simulink library "ScopeHandler"  (R2016b)
settings: Solver=VariableStepAuto  StartTime=0.0  StopTime=10.0  RelTol=1e-3
libraries: ConversionsLibrary x16, slrtlib x9, VariousLibrary x6
settings Model: Creator=Nathan  LastModifiedBy=march

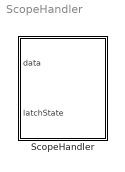
== system ScopeHandler ==
  ScopeHandler : Subsystem

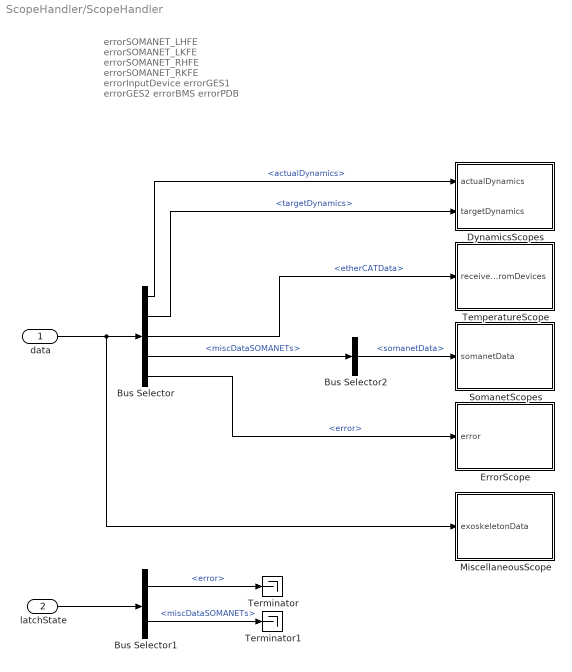
== system ScopeHandler/ScopeHandler ==
  note: errorSOMANET_LHFE
      | errorSOMANET_LKFE
      | errorSOMANET_RHFE
      | errorSOMANET_RKFE
      | errorInputDevice
      | errorGES1
      | errorGES2
      | errorBMS
      | errorPDB
  data : Inport  OutDataTypeStr=Bus: ExoskeletonData  BusOutputAsStruct=on
  latchState : Inport  Port=2  OutDataTypeStr=Bus: ExoskeletonData  BusOutputAsStruct=on
  Bus Selector : BusSelector  OutputSignals=actualDynamics,targetDynamics,etherCATData,miscDataSOMANETs,error
  Bus Selector1 : BusSelector  OutputSignals=error,miscDataSOMANETs
  Bus Selector2 : BusSelector  OutputSignals=somanetData
  DynamicsScopes : Subsystem
  ErrorScope : Subsystem
  MiscellaneousScope : Subsystem
  SomanetScopes : Subsystem
  TemperatureScope : Subsystem
  Terminator : Terminator
  Terminator1 : Terminator
  wires:
  Bus Selector2/1 -> SomanetScopes/1(somanetData)  "<somanetData>"
  Bus Selector/3 -> TemperatureScope/1(receivedFromDevices)  "<etherCATData>"
  Bus Selector/2 -> DynamicsScopes/2(targetDynamics)  "<targetDynamics>"
  Bus Selector/1 -> DynamicsScopes/1(actualDynamics)  "<actualDynamics>"
  Bus Selector/4 -> Bus Selector2/1  "<miscDataSOMANETs>"
  Bus Selector1/2 -> Terminator1/1  "<miscDataSOMANETs>"
  Bus Selector1/1 -> Terminator/1  "<error>"
  Bus Selector/5 -> ErrorScope/1(error)  "<error>"
  data/1 -> Bus Selector/1, MiscellaneousScope/1(exoskeletonData)
  latchState/1 -> Bus Selector1/1

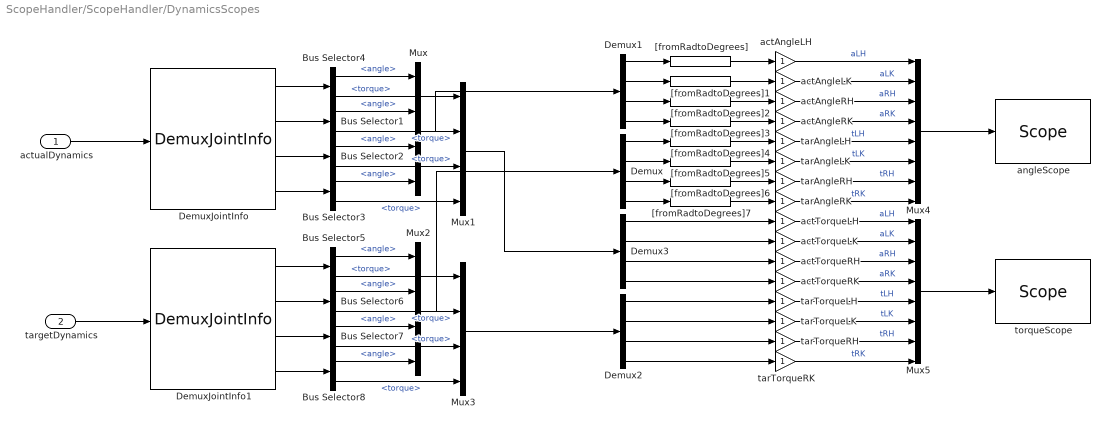
== system ScopeHandler/ScopeHandler/DynamicsScopes ==
  actualDynamics : Inport
  targetDynamics : Inport  Port=2
  Bus Selector{1..8} (8 alike) : BusSelector  OutputSignals=angle,torque
  Demux{,1..3} (4 alike) : Demux
  DemuxJointInfo : VariousLibrary/DemuxJointInfo
  DemuxJointInfo1 : VariousLibrary/DemuxJointInfo
  Mux{,1..3} (4 alike) : Mux
  Mux4 : Mux  Inputs=8
  Mux5 : Mux  Inputs=8
  [fromRadtoDegrees]{,1..7} (8 alike) : ConversionsLibrary/[fromRadtoDegrees]
  actAngleLH : Gain
  actAngleLK : Gain
  actAngleRH : Gain
  actAngleRK : Gain
  actTorqueLH : Gain
  actTorqueLK : Gain
  actTorqueRH : Gain
  actTorqueRK : Gain
  angleScope : slrtlib/Displays and Logging/Scope   scopeno=1  scopetype=Target  autostart=on  viewmode=Graphical rolling  formatstr='%15.6f'  grid=on  ylimits=[-180,180]  nosamples=2000  noprepostsamples=0  interleave=1  triggermode=FreeRun  triggersignal=1  trigsignalfromport=off  triggerlevel=0.0  triggerslope=Either  triggerscope=1  triggersample=0  filename=data.dat  mode=Lazy  writesize=512  autorestart=off  dynamicfilemode=off  maxwritefilesize=512*1024^2
  tarAngleLH : Gain
  tarAngleLK : Gain
  tarAngleRH : Gain
  tarAngleRK : Gain
  tarTorqueLH : Gain
  tarTorqueLK : Gain
  tarTorqueRH : Gain
  tarTorqueRK : Gain
  "torqueScope " : slrtlib/Displays and Logging/Scope   scopeno=2  scopetype=Target  autostart=on  viewmode=Graphical rolling  formatstr='%15.6f'  grid=on  ylimits=[-2.4,2.4]  nosamples=250  noprepostsamples=0  interleave=1  triggermode=FreeRun  triggersignal=1  trigsignalfromport=off  triggerlevel=0.0  triggerslope=Either  triggerscope=1  triggersample=0  filename=data.dat  mode=Lazy  writesize=512  autorestart=off  dynamicfilemode=off  maxwritefilesize=512*1024^2
  wires:
  Mux5/1 -> "torqueScope "/1
  Mux4/1 -> angleScope/1
  "[fromRadtoDegrees]7"/1 -> tarAngleRK/1
  "[fromRadtoDegrees]6"/1 -> tarAngleRH/1
  "[fromRadtoDegrees]5"/1 -> tarAngleLK/1
  "[fromRadtoDegrees]4"/1 -> tarAngleLH/1
  "[fromRadtoDegrees]3"/1 -> actAngleRK/1
  "[fromRadtoDegrees]2"/1 -> actAngleRH/1
  "[fromRadtoDegrees]1"/1 -> actAngleLK/1
  "[fromRadtoDegrees]"/1 -> actAngleLH/1
  tarTorqueRH/1 -> Mux5/7  "tRH"
  tarTorqueLK/1 -> Mux5/6  "tLK"
  tarTorqueLH/1 -> Mux5/5  "tLH"
  tarTorqueRK/1 -> Mux5/8  "tRK"
  Demux2/2 -> tarTorqueLK/1
  Demux2/1 -> tarTorqueLH/1
  Demux2/4 -> tarTorqueRK/1
  Demux2/3 -> tarTorqueRH/1
  actTorqueRK/1 -> Mux5/4  "aRK"
  actTorqueRH/1 -> Mux5/3  "aRH"
  actTorqueLK/1 -> Mux5/2  "aLK"
  actTorqueLH/1 -> Mux5/1  "aLH"
  Demux3/4 -> actTorqueRK/1
  Demux3/2 -> actTorqueLK/1
  Demux3/3 -> actTorqueRH/1
  Demux3/1 -> actTorqueLH/1
  tarAngleRK/1 -> Mux4/8  "tRK"
  tarAngleLH/1 -> Mux4/5  "tLH"
  tarAngleLK/1 -> Mux4/6  "tLK"
  tarAngleRH/1 -> Mux4/7  "tRH"
  Demux/2 -> "[fromRadtoDegrees]5"/1
  Demux/1 -> "[fromRadtoDegrees]4"/1
  Demux/3 -> "[fromRadtoDegrees]6"/1
  Demux/4 -> "[fromRadtoDegrees]7"/1
  actAngleRH/1 -> Mux4/3  "aRH"
  actAngleLH/1 -> Mux4/1  "aLH"
  actAngleLK/1 -> Mux4/2  "aLK"
  actAngleRK/1 -> Mux4/4  "aRK"
  Demux1/4 -> "[fromRadtoDegrees]3"/1
  Demux1/3 -> "[fromRadtoDegrees]2"/1
  Demux1/1 -> "[fromRadtoDegrees]"/1
  Demux1/2 -> "[fromRadtoDegrees]1"/1
  Mux3/1 -> Demux2/1
  Mux1/1 -> Demux3/1
  Mux2/1 -> Demux/1
  Mux/1 -> Demux1/1
  Bus Selector8/2 -> Mux3/4  "<torque>"
  Bus Selector8/1 -> Mux2/4  "<angle>"
  Bus Selector7/2 -> Mux3/3  "<torque>"
  Bus Selector7/1 -> Mux2/3  "<angle>"
  Bus Selector6/2 -> Mux3/2  "<torque>"
  Bus Selector6/1 -> Mux2/2  "<angle>"
  Bus Selector5/2 -> Mux3/1  "<torque>"
  Bus Selector5/1 -> Mux2/1  "<angle>"
  Bus Selector3/2 -> Mux1/4  "<torque>"
  Bus Selector3/1 -> Mux/4  "<angle>"
  Bus Selector2/2 -> Mux1/3  "<torque>"
  Bus Selector2/1 -> Mux/3  "<angle>"
  Bus Selector1/2 -> Mux1/2  "<torque>"
  Bus Selector1/1 -> Mux/2  "<angle>"
  Bus Selector4/2 -> Mux1/1  "<torque>"
  Bus Selector4/1 -> Mux/1  "<angle>"
  DemuxJointInfo1/3 -> Bus Selector7/1
  DemuxJointInfo1/4 -> Bus Selector8/1
  DemuxJointInfo1/1 -> Bus Selector5/1
  DemuxJointInfo1/2 -> Bus Selector6/1
  DemuxJointInfo/3 -> Bus Selector2/1
  DemuxJointInfo/1 -> Bus Selector4/1
  DemuxJointInfo/4 -> Bus Selector3/1
  DemuxJointInfo/2 -> Bus Selector1/1
  targetDynamics/1 -> DemuxJointInfo1/1
  actualDynamics/1 -> DemuxJointInfo/1

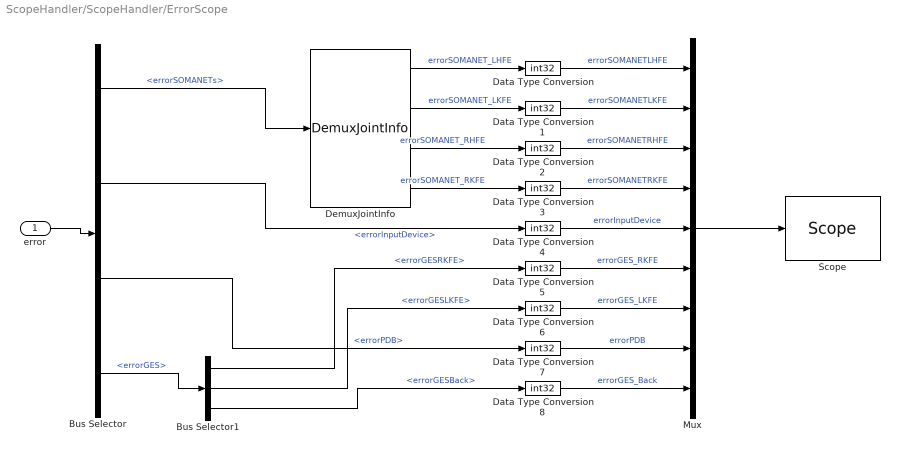
== system ScopeHandler/ScopeHandler/ErrorScope ==
  error : Inport
  Bus Selector : BusSelector  OutputSignals=errorSOMANETs,errorInputDevice,errorPowerElectronics.errorPDB,errorGES
  Bus Selector1 : BusSelector  OutputSignals=errorGESRKFE,errorGESLKFE,errorGESBack
  Data Type Conversion{,1..8} (9 alike) : DataTypeConversion  OutDataTypeStr=int32
  DemuxJointInfo : VariousLibrary/DemuxJointInfo
  Mux : Mux  Inputs=9
  "Scope " : slrtlib/Displays and Logging/Scope   scopeno=6  scopetype=Target  autostart=on  viewmode=Numerical  formatstr='%15.0f,%15.0f,%15.0f,%15.0f,%15.0f,%15.0f,%15.0f,%15.0f,%15.0f'  grid=on  ylimits=[0,0]  nosamples=250  noprepostsamples=0  interleave=1  triggermode=FreeRun  triggersignal=1  trigsignalfromport=off  triggerlevel=0.0  triggerslope=Either  triggerscope=1  triggersample=0  filename=data.dat  mode=Lazy  writesize=512  autorestart=off  dynamicfilemode=off  maxwritefilesize=512*1024^2
  wires:
  Bus Selector1/3 -> Data Type Conversion8/1  "<errorGESBack>"
  Bus Selector1/2 -> Data Type Conversion6/1  "<errorGESLKFE>"
  Bus Selector1/1 -> Data Type Conversion5/1  "<errorGESRKFE>"
  Data Type Conversion6/1 -> Mux/7  "errorGES_LKFE"
  Data Type Conversion5/1 -> Mux/6  "errorGES_RKFE"
  Data Type Conversion8/1 -> Mux/9  "errorGES_Back"
  Bus Selector/4 -> Bus Selector1/1  "<errorGES>"
  Data Type Conversion7/1 -> Mux/8  "errorPDB"
  Data Type Conversion4/1 -> Mux/5  "errorInputDevice"
  Data Type Conversion3/1 -> Mux/4  "errorSOMANETRKFE"
  Data Type Conversion2/1 -> Mux/3  "errorSOMANETRHFE"
  Data Type Conversion1/1 -> Mux/2  "errorSOMANETLKFE"
  Data Type Conversion/1 -> Mux/1  "errorSOMANETLHFE"
  Bus Selector/3 -> Data Type Conversion7/1  "<errorPDB>"
  Bus Selector/2 -> Data Type Conversion4/1  "<errorInputDevice>"
  Bus Selector/1 -> DemuxJointInfo/1  "<errorSOMANETs>"
  DemuxJointInfo/4 -> Data Type Conversion3/1  "errorSOMANET_RKFE"
  DemuxJointInfo/3 -> Data Type Conversion2/1  "errorSOMANET_RHFE"
  DemuxJointInfo/2 -> Data Type Conversion1/1  "errorSOMANET_LKFE"
  DemuxJointInfo/1 -> Data Type Conversion/1  "errorSOMANET_LHFE"
  Mux/1 -> "Scope "/1
  error/1 -> Bus Selector/1

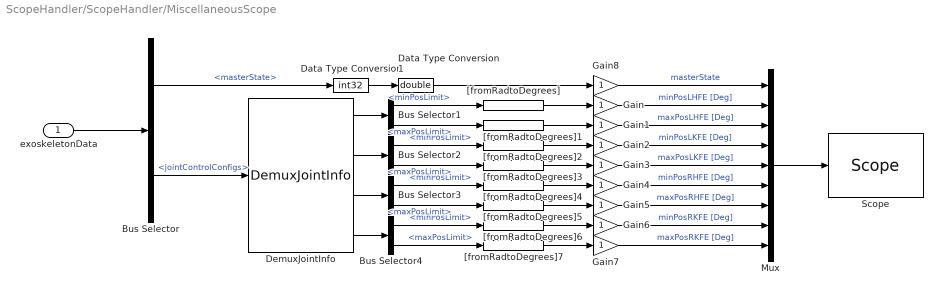
== system ScopeHandler/ScopeHandler/MiscellaneousScope ==
  exoskeletonData : Inport
  Bus Selector : BusSelector  OutputSignals=masterState,miscDataSOMANETs.jointControlConfigs
  Bus Selector{1..4} (4 alike) : BusSelector  OutputSignals=minPosLimit,maxPosLimit
  Data Type Conversion : DataTypeConversion  OutDataTypeStr=int32
  Data Type Conversion1 : DataTypeConversion  OutDataTypeStr=double
  DemuxJointInfo : VariousLibrary/DemuxJointInfo
  Gain{,1..8} (9 alike) : Gain
  Mux : Mux  Inputs=9
  "Scope " : slrtlib/Displays and Logging/Scope   scopeno=9  scopetype=Target  autostart=on  viewmode=Numerical  formatstr='%15.0f'  grid=on  ylimits=[0,0]  nosamples=250  noprepostsamples=0  interleave=1  triggermode=FreeRun  triggersignal=1  trigsignalfromport=off  triggerlevel=0.0  triggerslope=Either  triggerscope=1  triggersample=0  filename=data.dat  mode=Lazy  writesize=512  autorestart=off  dynamicfilemode=off  maxwritefilesize=512*1024^2
  [fromRadtoDegrees]{,1..7} (8 alike) : ConversionsLibrary/[fromRadtoDegrees]
  wires:
  Mux/1 -> "Scope "/1
  Gain5/1 -> Mux/7  "maxPosRHFE [Deg]"
  Gain3/1 -> Mux/5  "maxPosLKFE [Deg]"
  Gain2/1 -> Mux/4  "minPosLKFE [Deg]"
  Gain7/1 -> Mux/9  "maxPosRKFE [Deg]"
  Gain6/1 -> Mux/8  "minPosRKFE [Deg]"
  Gain/1 -> Mux/2  "minPosLHFE [Deg]"
  Gain4/1 -> Mux/6  "minPosRHFE [Deg]"
  Gain1/1 -> Mux/3  "maxPosLHFE [Deg]"
  Gain8/1 -> Mux/1  "masterState"
  Data Type Conversion1/1 -> Gain8/1
  Bus Selector/1 -> Data Type Conversion/1  "<masterState>"
  Data Type Conversion/1 -> Data Type Conversion1/1
  "[fromRadtoDegrees]7"/1 -> Gain7/1
  "[fromRadtoDegrees]6"/1 -> Gain6/1
  "[fromRadtoDegrees]5"/1 -> Gain5/1
  "[fromRadtoDegrees]4"/1 -> Gain4/1
  "[fromRadtoDegrees]3"/1 -> Gain3/1
  "[fromRadtoDegrees]2"/1 -> Gain2/1
  "[fromRadtoDegrees]1"/1 -> Gain1/1
  "[fromRadtoDegrees]"/1 -> Gain/1
  Bus Selector4/1 -> "[fromRadtoDegrees]6"/1  "<minPosLimit>"
  Bus Selector4/2 -> "[fromRadtoDegrees]7"/1  "<maxPosLimit>"
  Bus Selector3/2 -> "[fromRadtoDegrees]5"/1  "<maxPosLimit>"
  Bus Selector3/1 -> "[fromRadtoDegrees]4"/1  "<minPosLimit>"
  Bus Selector2/1 -> "[fromRadtoDegrees]2"/1  "<minPosLimit>"
  Bus Selector2/2 -> "[fromRadtoDegrees]3"/1  "<maxPosLimit>"
  Bus Selector1/2 -> "[fromRadtoDegrees]1"/1  "<maxPosLimit>"
  Bus Selector1/1 -> "[fromRadtoDegrees]"/1  "<minPosLimit>"
  DemuxJointInfo/3 -> Bus Selector3/1
  DemuxJointInfo/2 -> Bus Selector2/1
  DemuxJointInfo/4 -> Bus Selector4/1
  DemuxJointInfo/1 -> Bus Selector1/1
  Bus Selector/2 -> DemuxJointInfo/1  "<jointControlConfigs>"
  exoskeletonData/1 -> Bus Selector/1

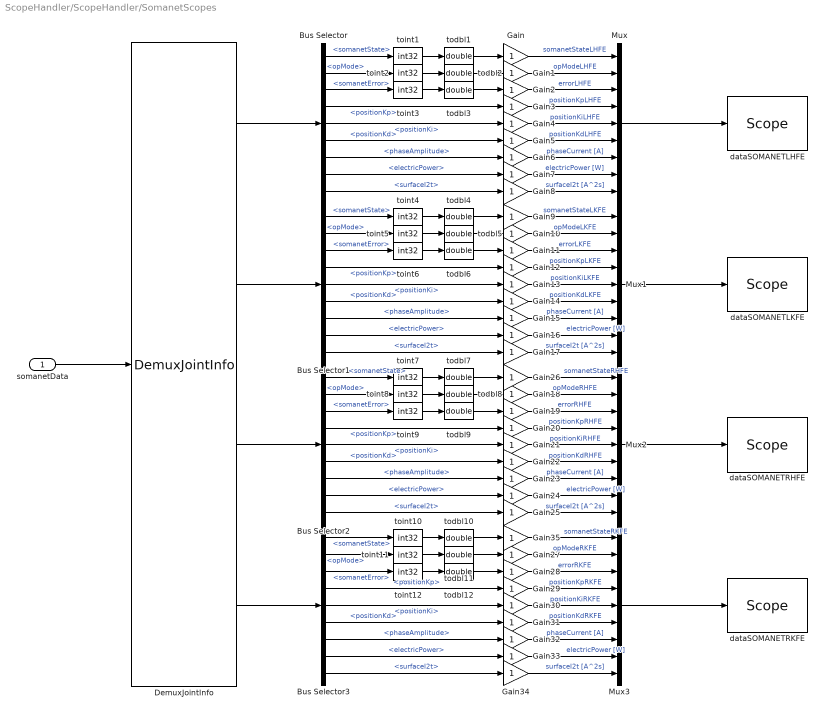
== system ScopeHandler/ScopeHandler/SomanetScopes ==
  somanetData : Inport
  Bus Selector{,1..3} (4 alike) : BusSelector  OutputSignals=somanetState,opMode,somanetError,positionKp,positionKi,positionKd,phaseAmplitude,electricPower,surfaceI2t
  DemuxJointInfo : VariousLibrary/DemuxJointInfo
  Gain{,1..35} (36 alike) : Gain
  Mux{,1..3} (4 alike) : Mux  Inputs=9
  dataSOMANETLHFE : slrtlib/Displays and Logging/Scope   scopeno=4  scopetype=Target  autostart=on  viewmode=Numerical  formatstr='%15.0f,%15.0f,%15.0f'  grid=on  ylimits=[0,0]  nosamples=250  noprepostsamples=0  interleave=1  triggermode=FreeRun  triggersignal=1  trigsignalfromport=off  triggerlevel=0.0  triggerslope=Either  triggerscope=1  triggersample=0  filename=data.dat  mode=Lazy  writesize=512  autorestart=off  dynamicfilemode=off  maxwritefilesize=512*1024^2
  "dataSOMANETLKFE " : slrtlib/Displays and Logging/Scope   scopeno=7  scopetype=Target  autostart=on  viewmode=Numerical  formatstr='%15.0f,%15.0f,%15.0f'  grid=on  ylimits=[0,0]  nosamples=250  noprepostsamples=0  interleave=1  triggermode=FreeRun  triggersignal=1  trigsignalfromport=off  triggerlevel=0.0  triggerslope=Either  triggerscope=1  triggersample=0  filename=data.dat  mode=Lazy  writesize=512  autorestart=off  dynamicfilemode=off  maxwritefilesize=512*1024^2
  dataSOMANETRHFE : slrtlib/Displays and Logging/Scope   scopeno=5  scopetype=Target  autostart=on  viewmode=Numerical  formatstr='%15.0f,%15.0f,%15.0f'  grid=on  ylimits=[0,0]  nosamples=250  noprepostsamples=0  interleave=1  triggermode=FreeRun  triggersignal=1  trigsignalfromport=off  triggerlevel=0.0  triggerslope=Either  triggerscope=1  triggersample=0  filename=data.dat  mode=Lazy  writesize=512  autorestart=off  dynamicfilemode=off  maxwritefilesize=512*1024^2
  dataSOMANETRKFE : slrtlib/Displays and Logging/Scope   scopeno=8  scopetype=Target  autostart=on  viewmode=Numerical  formatstr='%15.0f,%15.0f,%15.0f'  grid=on  ylimits=[0,0]  nosamples=250  noprepostsamples=0  interleave=1  triggermode=FreeRun  triggersignal=1  trigsignalfromport=off  triggerlevel=0.0  triggerslope=Either  triggerscope=1  triggersample=0  filename=data.dat  mode=Lazy  writesize=512  autorestart=off  dynamicfilemode=off  maxwritefilesize=512*1024^2
  todbl{1..12} (12 alike) : DataTypeConversion  OutDataTypeStr=double
  toint{1..12} (12 alike) : DataTypeConversion  OutDataTypeStr=int32
  wires:
  Bus Selector3/1 -> toint10/1  "<somanetState>"
  Bus Selector3/2 -> toint11/1  "<opMode>"
  Bus Selector3/3 -> toint12/1  "<somanetError>"
  Bus Selector2/3 -> toint9/1  "<somanetError>"
  Bus Selector2/2 -> toint8/1  "<opMode>"
  Bus Selector2/1 -> toint7/1  "<somanetState>"
  Bus Selector1/3 -> toint6/1  "<somanetError>"
  Bus Selector1/2 -> toint5/1  "<opMode>"
  Bus Selector1/1 -> toint4/1  "<somanetState>"
  todbl11/1 -> Gain27/1
  todbl12/1 -> Gain28/1
  todbl10/1 -> Gain35/1
  todbl9/1 -> Gain19/1
  todbl8/1 -> Gain18/1
  todbl7/1 -> Gain26/1
  todbl6/1 -> Gain11/1
  todbl5/1 -> Gain10/1
  todbl4/1 -> Gain9/1
  todbl3/1 -> Gain2/1
  todbl2/1 -> Gain1/1
  Bus Selector/2 -> toint2/1  "<opMode>"
  Bus Selector/3 -> toint3/1  "<somanetError>"
  toint12/1 -> todbl12/1
  toint11/1 -> todbl11/1
  toint10/1 -> todbl10/1
  toint9/1 -> todbl9/1
  toint8/1 -> todbl8/1
  toint7/1 -> todbl7/1
  toint6/1 -> todbl6/1
  toint5/1 -> todbl5/1
  toint4/1 -> todbl4/1
  toint3/1 -> todbl3/1
  toint2/1 -> todbl2/1
  todbl1/1 -> Gain/1
  Bus Selector/1 -> toint1/1  "<somanetState>"
  toint1/1 -> todbl1/1
  Mux/1 -> dataSOMANETLHFE/1
  Mux1/1 -> "dataSOMANETLKFE "/1
  Mux2/1 -> dataSOMANETRHFE/1
  Mux3/1 -> dataSOMANETRKFE/1
  Gain32/1 -> Mux3/7  "phaseCurrent [A]"
  Gain27/1 -> Mux3/2  "opModeRKFE"
  Gain29/1 -> Mux3/4  "positionKpRKFE"
  Gain35/1 -> Mux3/1  "somanetStateRKFE"
  Gain34/1 -> Mux3/9  "surfaceI2t [A^2s]"
  Gain33/1 -> Mux3/8  "electricPower [W]"
  Gain31/1 -> Mux3/6  "positionKdRKFE"
  Gain30/1 -> Mux3/5  "positionKiRKFE"
  Gain28/1 -> Mux3/3  "errorRKFE"
  Gain20/1 -> Mux2/4  "positionKpRHFE"
  Gain18/1 -> Mux2/2  "opModeRHFE"
  Gain25/1 -> Mux2/9  "surfaceI2t [A^2s]"
  Gain19/1 -> Mux2/3  "errorRHFE"
  Gain26/1 -> Mux2/1  "somanetStateRHFE"
  Gain24/1 -> Mux2/8  "electricPower [W]"
  Gain23/1 -> Mux2/7  "phaseCurrent [A]"
  Gain22/1 -> Mux2/6  "positionKdRHFE"
  Gain21/1 -> Mux2/5  "positionKiRHFE"
  Gain10/1 -> Mux1/2  "opModeLKFE"
  Gain9/1 -> Mux1/1  "somanetStateLKFE"
  Gain16/1 -> Mux1/8  "electricPower [W]"
  Gain12/1 -> Mux1/4  "positionKpLKFE"
  Gain15/1 -> Mux1/7  "phaseCurrent [A]"
  Gain11/1 -> Mux1/3  "errorLKFE"
  Gain14/1 -> Mux1/6  "positionKdLKFE"
  Gain13/1 -> Mux1/5  "positionKiLKFE"
  Gain17/1 -> Mux1/9  "surfaceI2t [A^2s]"
  Gain/1 -> Mux/1  "somanetStateLHFE"
  Gain4/1 -> Mux/5  "positionKiLHFE"
  Gain3/1 -> Mux/4  "positionKpLHFE"
  Gain5/1 -> Mux/6  "positionKdLHFE"
  Gain6/1 -> Mux/7  "phaseCurrent [A]"
  Gain7/1 -> Mux/8  "electricPower [W]"
  Gain1/1 -> Mux/2  "opModeLHFE"
  Gain2/1 -> Mux/3  "errorLHFE"
  Gain8/1 -> Mux/9  "surfaceI2t [A^2s]"
  Bus Selector3/8 -> Gain33/1  "<electricPower>"
  Bus Selector3/4 -> Gain29/1  "<positionKp>"
  Bus Selector3/9 -> Gain34/1  "<surfaceI2t>"
  Bus Selector3/7 -> Gain32/1  "<phaseAmplitude>"
  Bus Selector3/5 -> Gain30/1  "<positionKi>"
  Bus Selector3/6 -> Gain31/1  "<positionKd>"
  DemuxJointInfo/4 -> Bus Selector3/1
  Bus Selector2/8 -> Gain24/1  "<electricPower>"
  Bus Selector2/4 -> Gain20/1  "<positionKp>"
  Bus Selector2/9 -> Gain25/1  "<surfaceI2t>"
  Bus Selector2/7 -> Gain23/1  "<phaseAmplitude>"
  Bus Selector2/5 -> Gain21/1  "<positionKi>"
  Bus Selector2/6 -> Gain22/1  "<positionKd>"
  DemuxJointInfo/3 -> Bus Selector2/1
  Bus Selector1/8 -> Gain16/1  "<electricPower>"
  Bus Selector1/4 -> Gain12/1  "<positionKp>"
  Bus Selector1/9 -> Gain17/1  "<surfaceI2t>"
  Bus Selector1/7 -> Gain15/1  "<phaseAmplitude>"
  Bus Selector1/5 -> Gain13/1  "<positionKi>"
  Bus Selector1/6 -> Gain14/1  "<positionKd>"
  DemuxJointInfo/2 -> Bus Selector1/1
  Bus Selector/8 -> Gain7/1  "<electricPower>"
  Bus Selector/4 -> Gain3/1  "<positionKp>"
  Bus Selector/9 -> Gain8/1  "<surfaceI2t>"
  Bus Selector/7 -> Gain6/1  "<phaseAmplitude>"
  Bus Selector/5 -> Gain4/1  "<positionKi>"
  Bus Selector/6 -> Gain5/1  "<positionKd>"
  DemuxJointInfo/1 -> Bus Selector/1
  somanetData/1 -> DemuxJointInfo/1

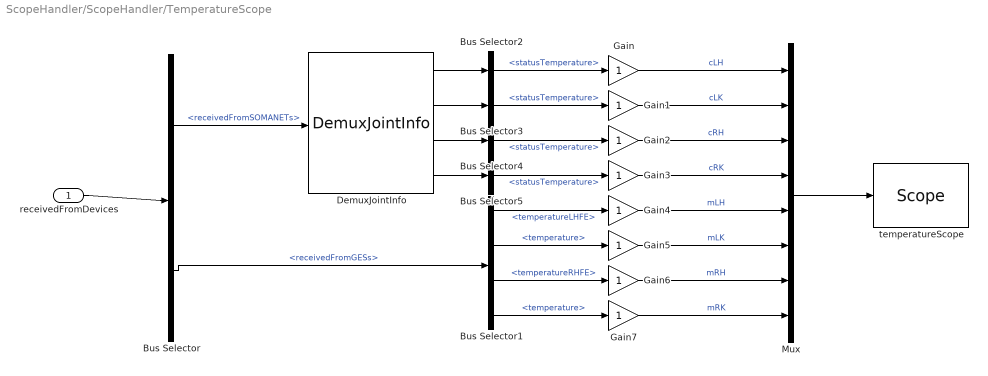
== system ScopeHandler/ScopeHandler/TemperatureScope ==
  receivedFromDevices : Inport  OutDataTypeStr=Bus: EtherCATData  PortDimensions=[1 4]
  Bus Selector : BusSelector  OutputSignals=receivedFromSOMANETs,receivedFromGESs
  Bus Selector1 : BusSelector  OutputSignals=receivedFromGESBack.temperatureLHFE,receivedFromGESLKFE.temperature,receivedFromGESBack.temperatureRHFE,receivedFromGESRKFE.temperature
  Bus Selector{2..5} (4 alike) : BusSelector  OutputSignals=statusTemperature
  DemuxJointInfo : VariousLibrary/DemuxJointInfo
  Gain{,1..7} (8 alike) : Gain
  Mux : Mux  Inputs=8
  temperatureScope : slrtlib/Displays and Logging/Scope   scopeno=3  scopetype=Target  autostart=on  viewmode=Graphical rolling  formatstr='%15.6f'  grid=on  ylimits=[20,140]  nosamples=2000  noprepostsamples=0  interleave=1  triggermode=FreeRun  triggersignal=1  trigsignalfromport=off  triggerlevel=0.0  triggerslope=Either  triggerscope=1  triggersample=0  filename=data.dat  mode=Lazy  writesize=512  autorestart=off  dynamicfilemode=off  maxwritefilesize=512*1024^2
  wires:
  Bus Selector5/1 -> Gain3/1  "<statusTemperature>"
  Bus Selector4/1 -> Gain2/1  "<statusTemperature>"
  Bus Selector3/1 -> Gain1/1  "<statusTemperature>"
  DemuxJointInfo/4 -> Bus Selector5/1
  DemuxJointInfo/3 -> Bus Selector4/1
  DemuxJointInfo/2 -> Bus Selector3/1
  Bus Selector2/1 -> Gain/1  "<statusTemperature>"
  DemuxJointInfo/1 -> Bus Selector2/1
  Mux/1 -> temperatureScope/1
  Gain7/1 -> Mux/8  "mRK"
  Gain6/1 -> Mux/7  "mRH"
  Gain5/1 -> Mux/6  "mLK"
  Gain4/1 -> Mux/5  "mLH"
  Gain3/1 -> Mux/4  "cRK"
  Gain2/1 -> Mux/3  "cRH"
  Gain1/1 -> Mux/2  "cLK"
  Gain/1 -> Mux/1  "cLH"
  Bus Selector1/1 -> Gain4/1  "<temperatureLHFE>"
  Bus Selector1/4 -> Gain7/1  "<temperature>"
  Bus Selector1/2 -> Gain5/1  "<temperature>"
  Bus Selector1/3 -> Gain6/1  "<temperatureRHFE>"
  Bus Selector/2 -> Bus Selector1/1  "<receivedFromGESs>"
  Bus Selector/1 -> DemuxJointInfo/1  "<receivedFromSOMANETs>"
  receivedFromDevices/1 -> Bus Selector/1
